simulink model "VDP"  (R2023b)
settings: Solver=VariableStepAuto  StartTime=0.0  StopTime=t(end)  RelTol=1e-3
values from neighbouring files (symbols this model uses):
  initial_conditions = [ ... (first row only)    [cheffer21_no_delay.m]
  params = [ ... (first row only)    [gois09_simulink.m]    (also in ryzhii14_simulink.m; sinoatrial_simulink.m; vdp_simulink.m)
settings Model: Creator=chukw  LastModifiedBy=chukw

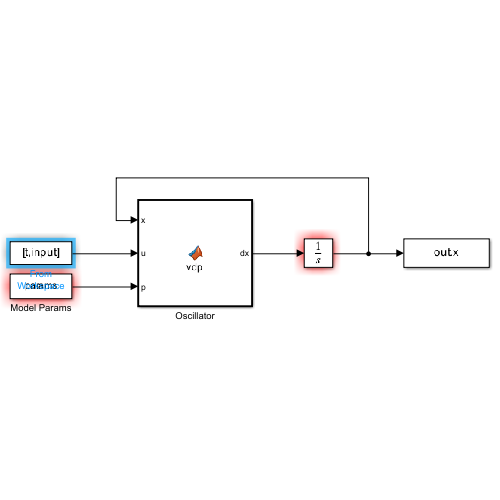
[thumbnail: Simulink's stored preview of the top-level diagram]
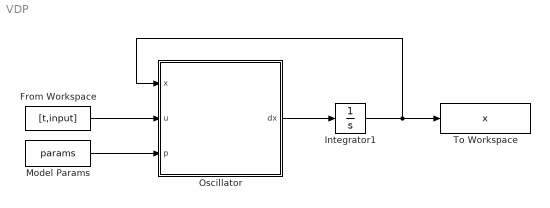
== system VDP ==
  From Workspace : FromWorkspace  VariableName=[t,input]
  Integrator1 : Integrator  InitialCondition=initial_conditions
  Model Params : Constant  Value=params
  Oscillator : MATLAB Function  TreatAsAtomicUnit=on
  To Workspace : ToWorkspace  VariableName=x  SampleTime=-1
  wires:
  From Workspace/1 -> Oscillator/2(u)
  Model Params/1 -> Oscillator/3(p)
  Integrator1/1 -> Oscillator/1(x), To Workspace/1
  Oscillator/1(dx) -> Integrator1/1

== matlab function VDP/Oscillator ==
  data: x input; u input; dx output; p input
function dx = vdp(x, u, p)
    eps = p(1);
    a = p(2);
    w = p(3);
    d = p(4);

    dx = zeros(2,1);
    dx(1) = x(2);
    dx(2) = eps*(1 - x(1)^2)*x(2) - ((w^2)*x(1)) + d*u;
end
